simulink model "gavin_mae490_Fuzzy"  (R2018b)
settings: Solver=VariableStepAuto  StartTime=0.0  StopTime=20  RelTol=1e-3
model workspace (MAT data in the model file):
  K = 1
  M = 1
undefined symbols (not defined in the file or in its folder): magnitude
libraries: fuzblock x1
settings Model: Creator=vojislav  LastModifiedBy=Nick

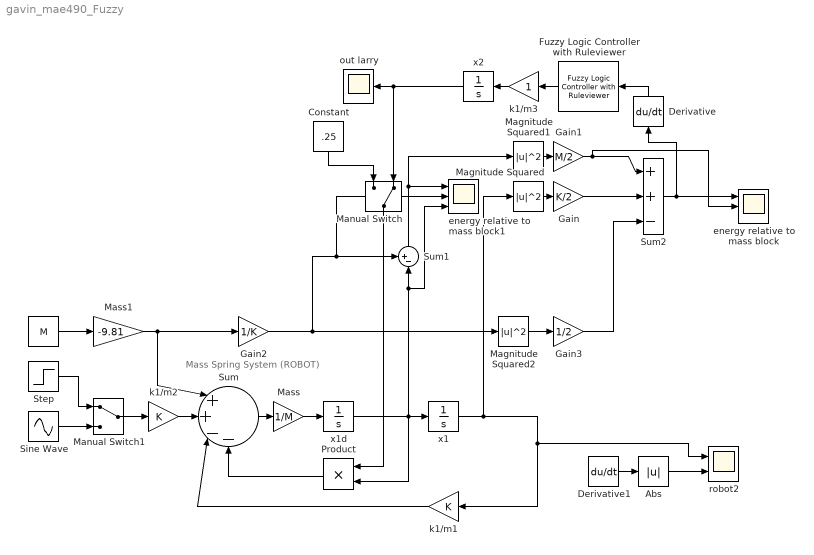
== system gavin_mae490_Fuzzy ==
  note: Mass Spring System (ROBOT)
  " " : Constant  Value=M
  Abs : Abs
  Constant : Constant  Value=.25
  Derivative : Derivative
  Derivative1 : Derivative
  Fuzzy Logic Controller with Ruleviewer : fuzblock/Fuzzy Logic  Controller  with Ruleviewer  fismatrix=larry  Ts=2
  Gain : Gain  Gain=K/2
  Gain1 : Gain  Gain=M/2
  Gain2 : Gain  Gain=1/K
  Gain3 : Gain  Gain=1/2
  Magnitude Squared : Math  Operator=magnitude^2  SaturateOnIntegerOverflow=on
  Magnitude Squared1 : Math  Operator=magnitude^2  SaturateOnIntegerOverflow=on
  Magnitude Squared2 : Math  Operator=magnitude^2  SaturateOnIntegerOverflow=on
  Manual Switch : ManualSwitch  CurrentSetting=0
  Manual Switch1 : ManualSwitch
  Mass : Gain  Gain=1/M
  Mass1 : Gain  Gain=-9.81
  Product : Product
  Sine Wave : Sin  SampleTime=0
  Step : Step  Time=2  SampleTime=0
  Sum : Sum  Inputs=|++--
  Sum1 : Sum  Inputs=+-|
  Sum2 : Sum  Inputs=++-
  energy relative to mass block : Scope  NumInputPorts=3
  energy relative to mass block1 : Scope  NumInputPorts=3
  k1/m1 : Gain  Gain=K
  k1/m2 : Gain  Gain=K
  k1/m3 : Gain
  "out larry " : Scope
  robot2 : Scope  NumInputPorts=2
  x1 : Integrator  InitialCondition=-10
  x1d : Integrator
  x2 : Integrator  InitialCondition=1
  wires:
  x1d/1 -> energy relative to mass block1/3, Sum1/2, Product/2, x1/1
  x1/1 -> Magnitude Squared/1, robot2/1, k1/m1/1
  Product/1 -> Sum/4
  Sum/1 -> Mass/1
  Mass/1 -> x1d/1
  " "/1 -> Mass1/1
  k1/m2/1 -> Sum/2
  k1/m1/1 -> Sum/3
  Magnitude Squared/1 -> Gain/1
  Sine Wave/1 -> Manual Switch1/2
  Magnitude Squared1/1 -> Gain1/1
  x2/1 -> Manual Switch/2, "out larry "/1
  Manual Switch/1 -> Product/1
  Constant/1 -> Manual Switch/1
  k1/m3/1 -> x2/1
  Fuzzy Logic Controller with Ruleviewer/1 -> k1/m3/1
  Step/1 -> Manual Switch1/1
  Manual Switch1/1 -> k1/m2/1
  Derivative/1 -> Fuzzy Logic Controller with Ruleviewer/1
  Mass1/1 -> Sum/1, Gain2/1
  Gain2/1 -> energy relative to mass block1/2, Sum1/1, Magnitude Squared2/1
  Magnitude Squared2/1 -> Gain3/1
  Sum2/1 -> Derivative/1, energy relative to mass block/1
  Sum1/1 -> Magnitude Squared1/1, energy relative to mass block1/1
  Gain/1 -> Sum2/2
  Gain1/1 -> energy relative to mass block/2, Sum2/1
  Gain3/1 -> Sum2/3
  Derivative1/1 -> Abs/1
  Abs/1 -> robot2/2
